simulink library "usask_tlm_lib"  (R2017b)
settings: Solver=ode45  StartTime=0.0  StopTime=10.0  RelTol=1e-3
undefined symbols (not defined in the file or in its folder): B, beta, d, K, L, lambda_1, m_E, m_G, mE_1, mE_2, mG_1, mG_2, nu, r1, r2, rho, T, Zc, Zc_1, Zc_2
libraries: usask_tlm_lib x6, transmission_lines x2
(part 4 of 4)

== system usask_tlm_lib/Tapered TLM Q1P2/G_1 ==
  note: Equation (17) from ven der Buhs et al. 2017
  F + P_1 : Inport
  Sum : Sum  Inputs=+------
  k = 1 : TransferFcn  Numerator=[m_G(1)*T 0]  Denominator=[T n(1)]
  k = 2 : TransferFcn  Numerator=[m_G(2)*T 0]  Denominator=[T n(2)]
  k = 3 : TransferFcn  Numerator=[m_G(3)*T 0]  Denominator=[T n(3)]
  k = 4 : TransferFcn  Numerator=[m_G(4)*T 0]  Denominator=[T n(4)]
  k = 5 : TransferFcn  Numerator=[m_G(5)*T 0]  Denominator=[T n(5)]
  k = 6 : TransferFcn  Numerator=[m_G(6)*T 0]  Denominator=[T n(6)]
  G : Outport
  wires:
  k = 6/1 -> Sum/7
  k = 5/1 -> Sum/6
  k = 4/1 -> Sum/5
  k = 2/1 -> Sum/3
  k = 1/1 -> Sum/2
  k = 3/1 -> Sum/4
  F + P_1/1 -> k = 3/1, k = 2/1, Sum/1, k = 1/1, k = 5/1, k = 6/1, k = 4/1
  Sum/1 -> G/1

== system usask_tlm_lib/Tapered TLM Q1P2/G_2 ==
  note: Equation (17) from ven der Buhs et al. 2017
  F + P_2 : Inport
  Sum : Sum  Inputs=+------
  k = 1 : TransferFcn  Numerator=[m_G(1)*T 0]  Denominator=[T n(1)]
  k = 2 : TransferFcn  Numerator=[m_G(2)*T 0]  Denominator=[T n(2)]
  k = 3 : TransferFcn  Numerator=[m_G(3)*T 0]  Denominator=[T n(3)]
  k = 4 : TransferFcn  Numerator=[m_G(4)*T 0]  Denominator=[T n(4)]
  k = 5 : TransferFcn  Numerator=[m_G(5)*T 0]  Denominator=[T n(5)]
  k = 6 : TransferFcn  Numerator=[m_G(6)*T 0]  Denominator=[T n(6)]
  G : Outport
  wires:
  k = 6/1 -> Sum/7
  k = 5/1 -> Sum/6
  k = 4/1 -> Sum/5
  k = 2/1 -> Sum/3
  k = 1/1 -> Sum/2
  k = 3/1 -> Sum/4
  F + P_2/1 -> k = 3/1, k = 2/1, Sum/1, k = 1/1, k = 5/1, k = 6/1, k = 4/1
  Sum/1 -> G/1

== system usask_tlm_lib/Tapered TLM Q1Q2/  Delay_2  ==
  G : Inport
  Transport Delay : TransportDelay  DelayTime=T_prime
  delay : Outport
  wires:
  Transport Delay/1 -> delay/1
  G/1 -> Transport Delay/1

== system usask_tlm_lib/Tapered TLM Q1Q2/Delay_1  ==
  G : Inport
  Transport Delay : TransportDelay  DelayTime=T_prime
  delay : Outport
  wires:
  Transport Delay/1 -> delay/1
  G/1 -> Transport Delay/1

== system usask_tlm_lib/Tapered TLM Q1Q2/E_1 ==
  note: Equation (14) from ven der Buhs et al. 2017
  Q_1 : Inport
  Gain : Gain  Gain=Z_c
  Sum : Sum  Inputs=++++++
  k = 1 : TransferFcn  Numerator=[m_E(1)]  Denominator=[T n(1)]
  k = 2 : TransferFcn  Numerator=[m_E(2)]  Denominator=[T n(2)]
  k = 3 : TransferFcn  Numerator=[m_E(3)]  Denominator=[T n(3)]
  k = 4 : TransferFcn  Numerator=[m_E(4)]  Denominator=[T n(4)]
  k = 5 : TransferFcn  Numerator=[m_E(5)]  Denominator=[T n(5)]
  k = 6 : TransferFcn  Numerator=[m_E(6)]  Denominator=[T n(6)]
  E : Outport
  wires:
  Q_1/1 -> k = 4/1, k = 5/1, k = 6/1, k = 3/1, k = 1/1, k = 2/1
  k = 6/1 -> Sum/6
  k = 5/1 -> Sum/5
  k = 4/1 -> Sum/4
  k = 3/1 -> Sum/3
  k = 2/1 -> Sum/2
  k = 1/1 -> Sum/1
  Sum/1 -> Gain/1
  Gain/1 -> E/1

== system usask_tlm_lib/Tapered TLM Q1Q2/E_2 ==
  note: Equation (14) from ven der Buhs et al. 2017
  Q_2 : Inport
  Gain : Gain  Gain=Z_c
  Sum : Sum  Inputs=++++++
  k = 1 : TransferFcn  Numerator=[m_E(1)]  Denominator=[T n(1)]
  k = 2 : TransferFcn  Numerator=[m_E(2)]  Denominator=[T n(2)]
  k = 3 : TransferFcn  Numerator=[m_E(3)]  Denominator=[T n(3)]
  k = 4 : TransferFcn  Numerator=[m_E(4)]  Denominator=[T n(4)]
  k = 5 : TransferFcn  Numerator=[m_E(5)]  Denominator=[T n(5)]
  k = 6 : TransferFcn  Numerator=[m_E(6)]  Denominator=[T n(6)]
  E : Outport
  wires:
  Q_2/1 -> k = 4/1, k = 5/1, k = 6/1, k = 3/1, k = 1/1, k = 2/1
  k = 6/1 -> Sum/6
  k = 5/1 -> Sum/5
  k = 4/1 -> Sum/4
  k = 3/1 -> Sum/3
  k = 2/1 -> Sum/2
  k = 1/1 -> Sum/1
  Sum/1 -> Gain/1
  Gain/1 -> E/1

== system usask_tlm_lib/Tapered TLM Q1Q2/F_1 ==
  note: Equation (15) from ven der Buhs et al. 2017
  Q_1 : Inport
  E : Inport  Port=2
  Gain : Gain  Gain=b
  Gain1 : Gain  Gain=Z_c
  Sum : Sum
  F : Outport
  wires:
  E/1 -> Gain/1
  Q_1/1 -> Gain1/1
  Sum/1 -> F/1
  Gain1/1 -> Sum/1
  Gain/1 -> Sum/2

== system usask_tlm_lib/Tapered TLM Q1Q2/F_2 ==
  note: Equation (15) from ven der Buhs et al. 2017
  E : Inport
  Q_2 : Inport  Port=2
  Gain : Gain  Gain=b
  Gain1 : Gain  Gain=Z_c
  Sum : Sum
  F : Outport
  wires:
  Gain/1 -> Sum/2
  Gain1/1 -> Sum/1
  Sum/1 -> F/1
  Q_2/1 -> Gain1/1
  E/1 -> Gain/1

== system usask_tlm_lib/Tapered TLM Q1Q2/G_1 ==
  note: Equation (17) from ven der Buhs et al. 2017
  F + P_1 : Inport
  Sum : Sum  Inputs=+------
  k = 1 : TransferFcn  Numerator=[m_G(1)*T 0]  Denominator=[T n(1)]
  k = 2 : TransferFcn  Numerator=[m_G(2)*T 0]  Denominator=[T n(2)]
  k = 3 : TransferFcn  Numerator=[m_G(3)*T 0]  Denominator=[T n(3)]
  k = 4 : TransferFcn  Numerator=[m_G(4)*T 0]  Denominator=[T n(4)]
  k = 5 : TransferFcn  Numerator=[m_G(5)*T 0]  Denominator=[T n(5)]
  k = 6 : TransferFcn  Numerator=[m_G(6)*T 0]  Denominator=[T n(6)]
  G : Outport
  wires:
  k = 6/1 -> Sum/7
  k = 5/1 -> Sum/6
  k = 4/1 -> Sum/5
  k = 2/1 -> Sum/3
  k = 1/1 -> Sum/2
  k = 3/1 -> Sum/4
  F + P_1/1 -> k = 3/1, k = 2/1, Sum/1, k = 1/1, k = 5/1, k = 6/1, k = 4/1
  Sum/1 -> G/1

== system usask_tlm_lib/Tapered TLM Q1Q2/G_2 ==
  note: Equation (17) from ven der Buhs et al. 2017
  F + P_2 : Inport
  Sum : Sum  Inputs=+------
  k = 1 : TransferFcn  Numerator=[m_G(1)*T 0]  Denominator=[T n(1)]
  k = 2 : TransferFcn  Numerator=[m_G(2)*T 0]  Denominator=[T n(2)]
  k = 3 : TransferFcn  Numerator=[m_G(3)*T 0]  Denominator=[T n(3)]
  k = 4 : TransferFcn  Numerator=[m_G(4)*T 0]  Denominator=[T n(4)]
  k = 5 : TransferFcn  Numerator=[m_G(5)*T 0]  Denominator=[T n(5)]
  k = 6 : TransferFcn  Numerator=[m_G(6)*T 0]  Denominator=[T n(6)]
  G : Outport
  wires:
  k = 6/1 -> Sum/7
  k = 5/1 -> Sum/6
  k = 4/1 -> Sum/5
  k = 2/1 -> Sum/3
  k = 1/1 -> Sum/2
  k = 3/1 -> Sum/4
  F + P_2/1 -> k = 3/1, k = 2/1, Sum/1, k = 1/1, k = 5/1, k = 6/1, k = 4/1
  Sum/1 -> G/1

== system usask_tlm_lib/Internal Blocks/Tapered TLM Base/Delay_1  ==
  G : Inport
  Transport Delay : TransportDelay  DelayTime=T
  delay : Outport
  wires:
  G/1 -> Transport Delay/1
  Transport Delay/1 -> delay/1

== system usask_tlm_lib/Internal Blocks/Tapered TLM Base/Delay_1 1 ==
  G : Inport
  Transport Delay : TransportDelay  DelayTime=T
  delay : Outport
  wires:
  G/1 -> Transport Delay/1
  Transport Delay/1 -> delay/1

== system usask_tlm_lib/Internal Blocks/Tapered TLM Base/E_1 ==
  Q_2 : Inport
  Gain : Gain  Gain=Zc
  Sum : Sum  Inputs=++++++
  k = 1 : TransferFcn  Numerator=[m_E(1)]  Denominator=[T n(1)]
  k = 2 : TransferFcn  Numerator=[m_E(2)]  Denominator=[T n(2)]
  k = 3 : TransferFcn  Numerator=[m_E(3)]  Denominator=[T n(3)]
  k = 4 : TransferFcn  Numerator=[m_E(4)]  Denominator=[T n(4)]
  k = 5 : TransferFcn  Numerator=[m_E(5)]  Denominator=[T n(5)]
  k = 6 : TransferFcn  Numerator=[m_E(6)]  Denominator=[T n(6)]
  E : Outport
  wires:
  Gain/1 -> E/1
  Sum/1 -> Gain/1
  k = 1/1 -> Sum/1
  k = 2/1 -> Sum/2
  k = 3/1 -> Sum/3
  k = 4/1 -> Sum/4
  k = 5/1 -> Sum/5
  k = 6/1 -> Sum/6
  Q_2/1 -> k = 2/1, k = 1/1, k = 3/1, k = 6/1, k = 5/1, k = 4/1

== system usask_tlm_lib/Internal Blocks/Tapered TLM Base/E_2 ==
  Q_2 : Inport
  Gain : Gain  Gain=Zc
  Sum : Sum  Inputs=++++++
  k = 1 : TransferFcn  Numerator=[m_E(1)]  Denominator=[T n(1)]
  k = 2 : TransferFcn  Numerator=[m_E(2)]  Denominator=[T n(2)]
  k = 3 : TransferFcn  Numerator=[m_E(3)]  Denominator=[T n(3)]
  k = 4 : TransferFcn  Numerator=[m_E(4)]  Denominator=[T n(4)]
  k = 5 : TransferFcn  Numerator=[m_E(5)]  Denominator=[T n(5)]
  k = 6 : TransferFcn  Numerator=[m_E(6)]  Denominator=[T n(6)]
  E : Outport
  wires:
  Gain/1 -> E/1
  Sum/1 -> Gain/1
  k = 1/1 -> Sum/1
  k = 2/1 -> Sum/2
  k = 3/1 -> Sum/3
  k = 4/1 -> Sum/4
  k = 5/1 -> Sum/5
  k = 6/1 -> Sum/6
  Q_2/1 -> k = 2/1, k = 1/1, k = 3/1, k = 6/1, k = 5/1, k = 4/1

== system usask_tlm_lib/Internal Blocks/Tapered TLM Base/F_3 ==
  Q_1 : Inport
  E : Inport  Port=2
  Gain : Gain  Gain=b
  Gain1 : Gain  Gain=Zc
  Gain2 : Gain  Gain=F_k
  Sum : Sum
  F : Outport
  wires:
  E/1 -> Gain/1
  Q_1/1 -> Gain1/1
  Sum/1 -> Gain2/1
  Gain1/1 -> Sum/1
  Gain/1 -> Sum/2
  Gain2/1 -> F/1

== system usask_tlm_lib/Internal Blocks/Tapered TLM Base/G_1 ==
  F + P_1 : Inport
  Gain : Gain  Gain=1-H_DC
  Sum : Sum  Inputs=+------
  k = 1 : TransferFcn  Numerator=[m_G(1)*T 0]  Denominator=[T n(1)]
  k = 2 : TransferFcn  Numerator=[m_G(2)*T 0]  Denominator=[T n(2)]
  k = 3 : TransferFcn  Numerator=[m_G(3)*T 0]  Denominator=[T n(3)]
  k = 4 : TransferFcn  Numerator=[m_G(4)*T 0]  Denominator=[T n(4)]
  k = 5 : TransferFcn  Numerator=[m_G(5)*T 0]  Denominator=[T n(5)]
  k = 6 : TransferFcn  Numerator=[m_G(6)*T 0]  Denominator=[T n(6)]
  G : Outport
  wires:
  Sum/1 -> Gain/1
  F + P_1/1 -> k = 4/1, k = 6/1, k = 5/1, k = 1/1, Sum/1, k = 2/1, k = 3/1
  k = 3/1 -> Sum/4
  k = 1/1 -> Sum/2
  k = 2/1 -> Sum/3
  k = 4/1 -> Sum/5
  k = 5/1 -> Sum/6
  k = 6/1 -> Sum/7
  Gain/1 -> G/1

== system usask_tlm_lib/Internal Blocks/Tapered TLM Base/G_3 ==
  F + P_1 : Inport
  Gain : Gain  Gain=1-H_DC
  Sum : Sum  Inputs=+------
  k = 1 : TransferFcn  Numerator=[m_G(1)*T 0]  Denominator=[T n(1)]
  k = 2 : TransferFcn  Numerator=[m_G(2)*T 0]  Denominator=[T n(2)]
  k = 3 : TransferFcn  Numerator=[m_G(3)*T 0]  Denominator=[T n(3)]
  k = 4 : TransferFcn  Numerator=[m_G(4)*T 0]  Denominator=[T n(4)]
  k = 5 : TransferFcn  Numerator=[m_G(5)*T 0]  Denominator=[T n(5)]
  k = 6 : TransferFcn  Numerator=[m_G(6)*T 0]  Denominator=[T n(6)]
  G : Outport
  wires:
  Sum/1 -> Gain/1
  F + P_1/1 -> k = 4/1, k = 6/1, k = 5/1, k = 1/1, Sum/1, k = 2/1, k = 3/1
  k = 3/1 -> Sum/4
  k = 1/1 -> Sum/2
  k = 2/1 -> Sum/3
  k = 4/1 -> Sum/5
  k = 5/1 -> Sum/6
  k = 6/1 -> Sum/7
  Gain/1 -> G/1

== system usask_tlm_lib/Internal Blocks/Tapered TLM Base/H_1 ==
  in : Inport
  Add1 : Sum  Inputs=+-+
  Add2 : Sum  Inputs=-+
  Gain2 : Gain  Gain=H_a
  Gain3 : Gain  Gain=H_b
  Gain5 : Gain  Gain=(H_b-H_a)/T
  Integrator1 : Integrator
  Integrator2 : Integrator
  Integrator3 : Integrator
  Transport Delay1 : TransportDelay  DelayTime=T
  out : Outport
  wires:
  Add2/1 -> Gain5/1
  Integrator1/1 -> Add2/1
  Gain5/1 -> Add1/3
  Gain3/1 -> Add1/2
  Add1/1 -> out/1  "S"
  Gain2/1 -> Add1/1
  Transport Delay1/1 -> Gain3/1, Integrator1/1
  Integrator3/1 -> Add2/2
  Integrator2/1 -> Transport Delay1/1, Gain2/1, Integrator3/1
  in/1 -> Integrator2/1

== system usask_tlm_lib/Internal Blocks/Tapered TLM Base/H_2 ==
  in : Inport
  Add1 : Sum  Inputs=+-+
  Add2 : Sum  Inputs=-+
  Gain2 : Gain  Gain=H_a
  Gain3 : Gain  Gain=H_b
  Gain5 : Gain  Gain=(H_b-H_a)/T
  Integrator1 : Integrator
  Integrator2 : Integrator
  Integrator3 : Integrator
  Transport Delay1 : TransportDelay  DelayTime=T
  out : Outport
  wires:
  Add2/1 -> Gain5/1
  Integrator1/1 -> Add2/1
  Gain5/1 -> Add1/3
  Gain3/1 -> Add1/2
  Add1/1 -> out/1  "S"
  Gain2/1 -> Add1/1
  Transport Delay1/1 -> Gain3/1, Integrator1/1
  Integrator3/1 -> Add2/2
  Integrator2/1 -> Transport Delay1/1, Gain2/1, Integrator3/1
  in/1 -> Integrator2/1

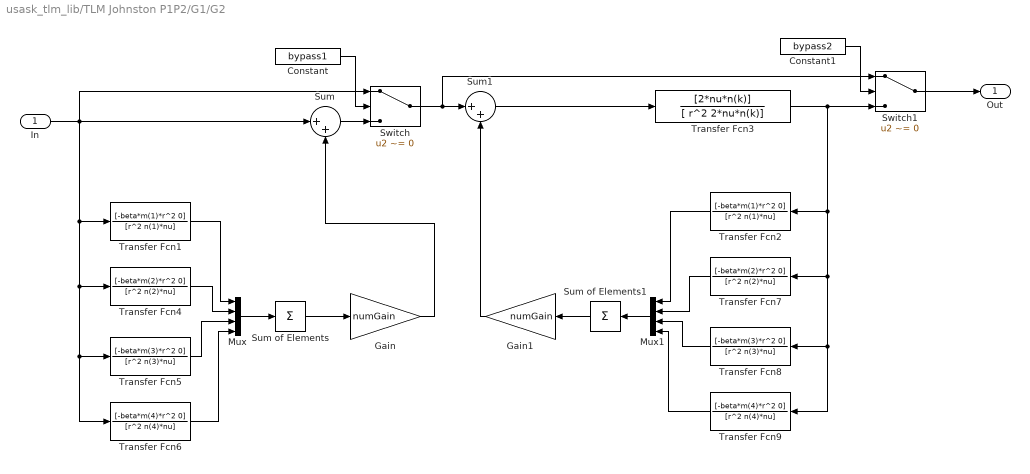
== system usask_tlm_lib/TLM Johnston P1P2/G1/G2 ==
  In : Inport
  Constant : Constant  Value=bypass1
  Constant1 : Constant  Value=bypass2
  Gain : Gain  Gain=numGain
  Gain1 : Gain  Gain=numGain
  Mux : Mux
  Mux1 : Mux
  Sum : Sum  Inputs=|++
  Sum of Elements : Sum  Inputs=+
  Sum of Elements1 : Sum  Inputs=+
  Sum1 : Sum  Inputs=|++
  Switch : Switch  Criteria=u2 ~= 0
  Switch1 : Switch  Criteria=u2 ~= 0
  Transfer Fcn1 : TransferFcn  Numerator=[-beta*m(1)*r^2 0]  Denominator=[r^2 n(1)*nu]
  Transfer Fcn2 : TransferFcn  Numerator=[-beta*m(1)*r^2 0]  Denominator=[r^2 n(1)*nu]
  Transfer Fcn3 : TransferFcn  Numerator=[2*nu*n(k)]  Denominator=[ r^2 2*nu*n(k)]
  Transfer Fcn4 : TransferFcn  Numerator=[-beta*m(2)*r^2 0]  Denominator=[r^2 n(2)*nu]
  Transfer Fcn5 : TransferFcn  Numerator=[-beta*m(3)*r^2 0]  Denominator=[r^2 n(3)*nu]
  Transfer Fcn6 : TransferFcn  Numerator=[-beta*m(4)*r^2 0]  Denominator=[r^2 n(4)*nu]
  Transfer Fcn7 : TransferFcn  Numerator=[-beta*m(2)*r^2 0]  Denominator=[r^2 n(2)*nu]
  Transfer Fcn8 : TransferFcn  Numerator=[-beta*m(3)*r^2 0]  Denominator=[r^2 n(3)*nu]
  Transfer Fcn9 : TransferFcn  Numerator=[-beta*m(4)*r^2 0]  Denominator=[r^2 n(4)*nu]
  Out : Outport
  wires:
  Sum1/1 -> Transfer Fcn3/1
  Gain1/1 -> Sum1/2
  Gain/1 -> Sum/2
  Mux1/1 -> Sum of Elements1/1
  Transfer Fcn9/1 -> Mux1/4
  Transfer Fcn2/1 -> Mux1/1
  Transfer Fcn8/1 -> Mux1/3
  Transfer Fcn7/1 -> Mux1/2
  Sum of Elements1/1 -> Gain1/1
  Mux/1 -> Sum of Elements/1
  Transfer Fcn6/1 -> Mux/4
  Transfer Fcn1/1 -> Mux/1
  Transfer Fcn5/1 -> Mux/3
  Transfer Fcn4/1 -> Mux/2
  Constant1/1 -> Switch1/2
  Constant/1 -> Switch/2
  Switch1/1 -> Out/1
  Switch/1 -> Sum1/1, Switch1/1
  Sum/1 -> Switch/3
  Transfer Fcn3/1 -> Switch1/3, Transfer Fcn2/1, Transfer Fcn7/1, Transfer Fcn8/1, Transfer Fcn9/1
  Sum of Elements/1 -> Gain/1
  In/1 -> Sum/1, Transfer Fcn1/1, Transfer Fcn4/1, Transfer Fcn5/1, Transfer Fcn6/1, Switch/1

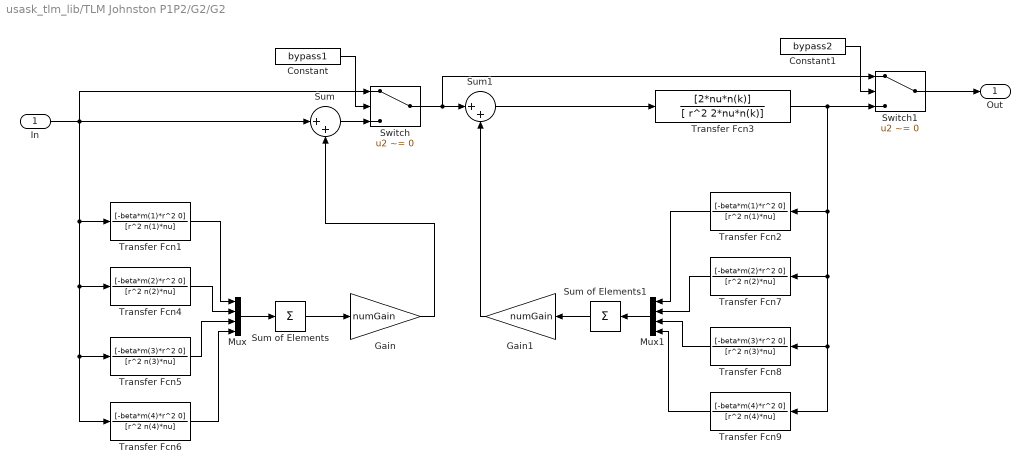
== system usask_tlm_lib/TLM Johnston P1P2/G2/G2 ==
  In : Inport
  Constant : Constant  Value=bypass1
  Constant1 : Constant  Value=bypass2
  Gain : Gain  Gain=numGain
  Gain1 : Gain  Gain=numGain
  Mux : Mux
  Mux1 : Mux
  Sum : Sum  Inputs=|++
  Sum of Elements : Sum  Inputs=+
  Sum of Elements1 : Sum  Inputs=+
  Sum1 : Sum  Inputs=|++
  Switch : Switch  Criteria=u2 ~= 0
  Switch1 : Switch  Criteria=u2 ~= 0
  Transfer Fcn1 : TransferFcn  Numerator=[-beta*m(1)*r^2 0]  Denominator=[r^2 n(1)*nu]
  Transfer Fcn2 : TransferFcn  Numerator=[-beta*m(1)*r^2 0]  Denominator=[r^2 n(1)*nu]
  Transfer Fcn3 : TransferFcn  Numerator=[2*nu*n(k)]  Denominator=[ r^2 2*nu*n(k)]
  Transfer Fcn4 : TransferFcn  Numerator=[-beta*m(2)*r^2 0]  Denominator=[r^2 n(2)*nu]
  Transfer Fcn5 : TransferFcn  Numerator=[-beta*m(3)*r^2 0]  Denominator=[r^2 n(3)*nu]
  Transfer Fcn6 : TransferFcn  Numerator=[-beta*m(4)*r^2 0]  Denominator=[r^2 n(4)*nu]
  Transfer Fcn7 : TransferFcn  Numerator=[-beta*m(2)*r^2 0]  Denominator=[r^2 n(2)*nu]
  Transfer Fcn8 : TransferFcn  Numerator=[-beta*m(3)*r^2 0]  Denominator=[r^2 n(3)*nu]
  Transfer Fcn9 : TransferFcn  Numerator=[-beta*m(4)*r^2 0]  Denominator=[r^2 n(4)*nu]
  Out : Outport
  wires:
  Sum1/1 -> Transfer Fcn3/1
  Gain1/1 -> Sum1/2
  Gain/1 -> Sum/2
  Mux1/1 -> Sum of Elements1/1
  Transfer Fcn9/1 -> Mux1/4
  Transfer Fcn2/1 -> Mux1/1
  Transfer Fcn8/1 -> Mux1/3
  Transfer Fcn7/1 -> Mux1/2
  Sum of Elements1/1 -> Gain1/1
  Mux/1 -> Sum of Elements/1
  Transfer Fcn6/1 -> Mux/4
  Transfer Fcn1/1 -> Mux/1
  Transfer Fcn5/1 -> Mux/3
  Transfer Fcn4/1 -> Mux/2
  Constant1/1 -> Switch1/2
  Constant/1 -> Switch/2
  Switch1/1 -> Out/1
  Switch/1 -> Sum1/1, Switch1/1
  Sum/1 -> Switch/3
  Transfer Fcn3/1 -> Switch1/3, Transfer Fcn2/1, Transfer Fcn7/1, Transfer Fcn8/1, Transfer Fcn9/1
  Sum of Elements/1 -> Gain/1
  In/1 -> Sum/1, Transfer Fcn1/1, Transfer Fcn4/1, Transfer Fcn5/1, Transfer Fcn6/1, Switch/1

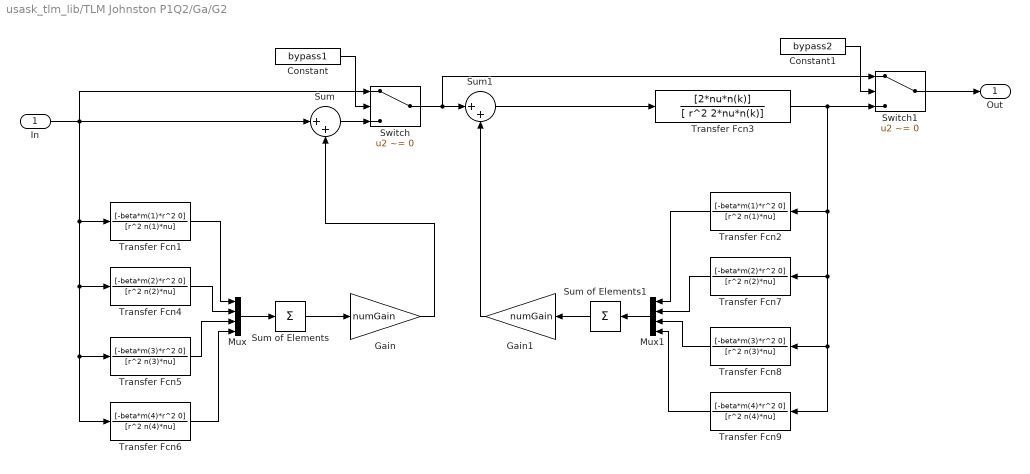
== system usask_tlm_lib/TLM Johnston P1Q2/Ga/G2 ==
  In : Inport
  Constant : Constant  Value=bypass1
  Constant1 : Constant  Value=bypass2
  Gain : Gain  Gain=numGain
  Gain1 : Gain  Gain=numGain
  Mux : Mux
  Mux1 : Mux
  Sum : Sum  Inputs=|++
  Sum of Elements : Sum  Inputs=+
  Sum of Elements1 : Sum  Inputs=+
  Sum1 : Sum  Inputs=|++
  Switch : Switch  Criteria=u2 ~= 0
  Switch1 : Switch  Criteria=u2 ~= 0
  Transfer Fcn1 : TransferFcn  Numerator=[-beta*m(1)*r^2 0]  Denominator=[r^2 n(1)*nu]
  Transfer Fcn2 : TransferFcn  Numerator=[-beta*m(1)*r^2 0]  Denominator=[r^2 n(1)*nu]
  Transfer Fcn3 : TransferFcn  Numerator=[2*nu*n(k)]  Denominator=[ r^2 2*nu*n(k)]
  Transfer Fcn4 : TransferFcn  Numerator=[-beta*m(2)*r^2 0]  Denominator=[r^2 n(2)*nu]
  Transfer Fcn5 : TransferFcn  Numerator=[-beta*m(3)*r^2 0]  Denominator=[r^2 n(3)*nu]
  Transfer Fcn6 : TransferFcn  Numerator=[-beta*m(4)*r^2 0]  Denominator=[r^2 n(4)*nu]
  Transfer Fcn7 : TransferFcn  Numerator=[-beta*m(2)*r^2 0]  Denominator=[r^2 n(2)*nu]
  Transfer Fcn8 : TransferFcn  Numerator=[-beta*m(3)*r^2 0]  Denominator=[r^2 n(3)*nu]
  Transfer Fcn9 : TransferFcn  Numerator=[-beta*m(4)*r^2 0]  Denominator=[r^2 n(4)*nu]
  Out : Outport
  wires:
  In/1 -> Switch/1, Transfer Fcn6/1, Transfer Fcn5/1, Transfer Fcn4/1, Transfer Fcn1/1, Sum/1
  Sum of Elements/1 -> Gain/1
  Transfer Fcn3/1 -> Transfer Fcn9/1, Transfer Fcn8/1, Transfer Fcn7/1, Transfer Fcn2/1, Switch1/3
  Sum/1 -> Switch/3
  Switch/1 -> Switch1/1, Sum1/1
  Switch1/1 -> Out/1
  Constant/1 -> Switch/2
  Constant1/1 -> Switch1/2
  Transfer Fcn4/1 -> Mux/2
  Transfer Fcn5/1 -> Mux/3
  Transfer Fcn1/1 -> Mux/1
  Transfer Fcn6/1 -> Mux/4
  Mux/1 -> Sum of Elements/1
  Sum of Elements1/1 -> Gain1/1
  Transfer Fcn7/1 -> Mux1/2
  Transfer Fcn8/1 -> Mux1/3
  Transfer Fcn2/1 -> Mux1/1
  Transfer Fcn9/1 -> Mux1/4
  Mux1/1 -> Sum of Elements1/1
  Gain/1 -> Sum/2
  Gain1/1 -> Sum1/2
  Sum1/1 -> Transfer Fcn3/1

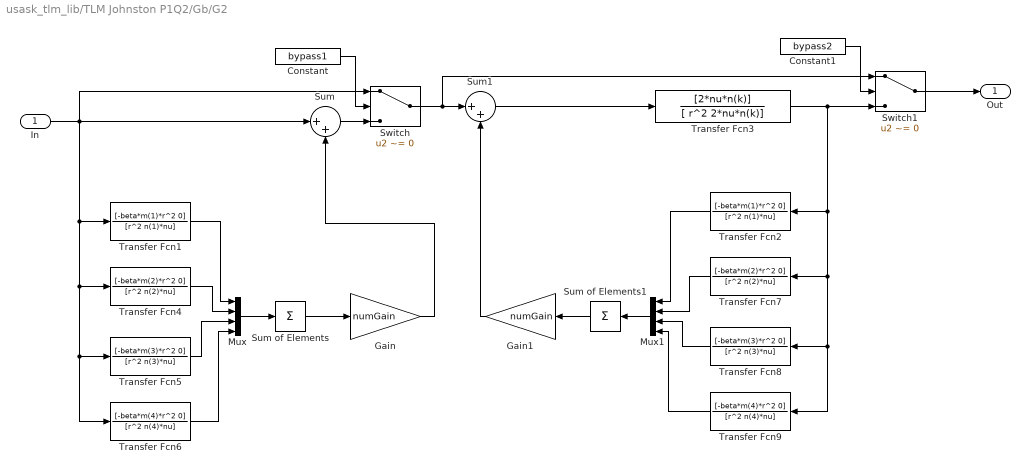
== system usask_tlm_lib/TLM Johnston P1Q2/Gb/G2 ==
  In : Inport
  Constant : Constant  Value=bypass1
  Constant1 : Constant  Value=bypass2
  Gain : Gain  Gain=numGain
  Gain1 : Gain  Gain=numGain
  Mux : Mux
  Mux1 : Mux
  Sum : Sum  Inputs=|++
  Sum of Elements : Sum  Inputs=+
  Sum of Elements1 : Sum  Inputs=+
  Sum1 : Sum  Inputs=|++
  Switch : Switch  Criteria=u2 ~= 0
  Switch1 : Switch  Criteria=u2 ~= 0
  Transfer Fcn1 : TransferFcn  Numerator=[-beta*m(1)*r^2 0]  Denominator=[r^2 n(1)*nu]
  Transfer Fcn2 : TransferFcn  Numerator=[-beta*m(1)*r^2 0]  Denominator=[r^2 n(1)*nu]
  Transfer Fcn3 : TransferFcn  Numerator=[2*nu*n(k)]  Denominator=[ r^2 2*nu*n(k)]
  Transfer Fcn4 : TransferFcn  Numerator=[-beta*m(2)*r^2 0]  Denominator=[r^2 n(2)*nu]
  Transfer Fcn5 : TransferFcn  Numerator=[-beta*m(3)*r^2 0]  Denominator=[r^2 n(3)*nu]
  Transfer Fcn6 : TransferFcn  Numerator=[-beta*m(4)*r^2 0]  Denominator=[r^2 n(4)*nu]
  Transfer Fcn7 : TransferFcn  Numerator=[-beta*m(2)*r^2 0]  Denominator=[r^2 n(2)*nu]
  Transfer Fcn8 : TransferFcn  Numerator=[-beta*m(3)*r^2 0]  Denominator=[r^2 n(3)*nu]
  Transfer Fcn9 : TransferFcn  Numerator=[-beta*m(4)*r^2 0]  Denominator=[r^2 n(4)*nu]
  Out : Outport
  wires:
  In/1 -> Switch/1, Transfer Fcn6/1, Transfer Fcn5/1, Transfer Fcn4/1, Transfer Fcn1/1, Sum/1
  Sum of Elements/1 -> Gain/1
  Transfer Fcn3/1 -> Transfer Fcn9/1, Transfer Fcn8/1, Transfer Fcn7/1, Transfer Fcn2/1, Switch1/3
  Sum/1 -> Switch/3
  Switch/1 -> Switch1/1, Sum1/1
  Switch1/1 -> Out/1
  Constant/1 -> Switch/2
  Constant1/1 -> Switch1/2
  Transfer Fcn4/1 -> Mux/2
  Transfer Fcn5/1 -> Mux/3
  Transfer Fcn1/1 -> Mux/1
  Transfer Fcn6/1 -> Mux/4
  Mux/1 -> Sum of Elements/1
  Sum of Elements1/1 -> Gain1/1
  Transfer Fcn7/1 -> Mux1/2
  Transfer Fcn8/1 -> Mux1/3
  Transfer Fcn2/1 -> Mux1/1
  Transfer Fcn9/1 -> Mux1/4
  Mux1/1 -> Sum of Elements1/1
  Gain/1 -> Sum/2
  Gain1/1 -> Sum1/2
  Sum1/1 -> Transfer Fcn3/1

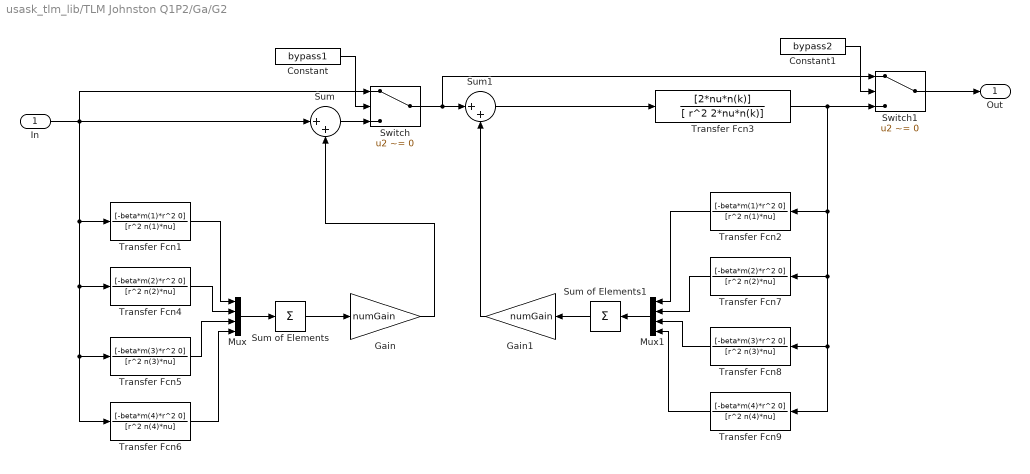
== system usask_tlm_lib/TLM Johnston Q1P2/Ga/G2 ==
  In : Inport
  Constant : Constant  Value=bypass1
  Constant1 : Constant  Value=bypass2
  Gain : Gain  Gain=numGain
  Gain1 : Gain  Gain=numGain
  Mux : Mux
  Mux1 : Mux
  Sum : Sum  Inputs=|++
  Sum of Elements : Sum  Inputs=+
  Sum of Elements1 : Sum  Inputs=+
  Sum1 : Sum  Inputs=|++
  Switch : Switch  Criteria=u2 ~= 0
  Switch1 : Switch  Criteria=u2 ~= 0
  Transfer Fcn1 : TransferFcn  Numerator=[-beta*m(1)*r^2 0]  Denominator=[r^2 n(1)*nu]
  Transfer Fcn2 : TransferFcn  Numerator=[-beta*m(1)*r^2 0]  Denominator=[r^2 n(1)*nu]
  Transfer Fcn3 : TransferFcn  Numerator=[2*nu*n(k)]  Denominator=[ r^2 2*nu*n(k)]
  Transfer Fcn4 : TransferFcn  Numerator=[-beta*m(2)*r^2 0]  Denominator=[r^2 n(2)*nu]
  Transfer Fcn5 : TransferFcn  Numerator=[-beta*m(3)*r^2 0]  Denominator=[r^2 n(3)*nu]
  Transfer Fcn6 : TransferFcn  Numerator=[-beta*m(4)*r^2 0]  Denominator=[r^2 n(4)*nu]
  Transfer Fcn7 : TransferFcn  Numerator=[-beta*m(2)*r^2 0]  Denominator=[r^2 n(2)*nu]
  Transfer Fcn8 : TransferFcn  Numerator=[-beta*m(3)*r^2 0]  Denominator=[r^2 n(3)*nu]
  Transfer Fcn9 : TransferFcn  Numerator=[-beta*m(4)*r^2 0]  Denominator=[r^2 n(4)*nu]
  Out : Outport
  wires:
  In/1 -> Switch/1, Transfer Fcn6/1, Transfer Fcn5/1, Transfer Fcn4/1, Transfer Fcn1/1, Sum/1
  Sum of Elements/1 -> Gain/1
  Transfer Fcn3/1 -> Transfer Fcn9/1, Transfer Fcn8/1, Transfer Fcn7/1, Transfer Fcn2/1, Switch1/3
  Sum/1 -> Switch/3
  Switch/1 -> Switch1/1, Sum1/1
  Switch1/1 -> Out/1
  Constant/1 -> Switch/2
  Constant1/1 -> Switch1/2
  Transfer Fcn4/1 -> Mux/2
  Transfer Fcn5/1 -> Mux/3
  Transfer Fcn1/1 -> Mux/1
  Transfer Fcn6/1 -> Mux/4
  Mux/1 -> Sum of Elements/1
  Sum of Elements1/1 -> Gain1/1
  Transfer Fcn7/1 -> Mux1/2
  Transfer Fcn8/1 -> Mux1/3
  Transfer Fcn2/1 -> Mux1/1
  Transfer Fcn9/1 -> Mux1/4
  Mux1/1 -> Sum of Elements1/1
  Gain/1 -> Sum/2
  Gain1/1 -> Sum1/2
  Sum1/1 -> Transfer Fcn3/1

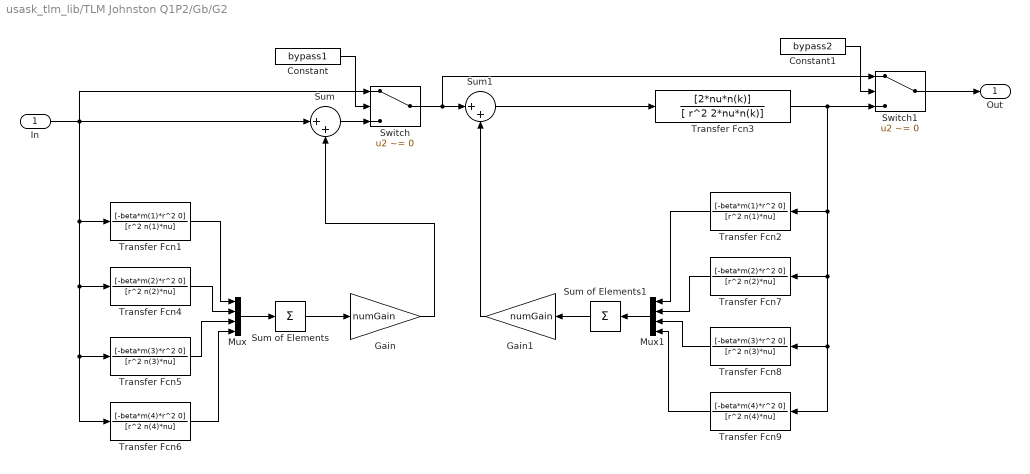
== system usask_tlm_lib/TLM Johnston Q1P2/Gb/G2 ==
  In : Inport
  Constant : Constant  Value=bypass1
  Constant1 : Constant  Value=bypass2
  Gain : Gain  Gain=numGain
  Gain1 : Gain  Gain=numGain
  Mux : Mux
  Mux1 : Mux
  Sum : Sum  Inputs=|++
  Sum of Elements : Sum  Inputs=+
  Sum of Elements1 : Sum  Inputs=+
  Sum1 : Sum  Inputs=|++
  Switch : Switch  Criteria=u2 ~= 0
  Switch1 : Switch  Criteria=u2 ~= 0
  Transfer Fcn1 : TransferFcn  Numerator=[-beta*m(1)*r^2 0]  Denominator=[r^2 n(1)*nu]
  Transfer Fcn2 : TransferFcn  Numerator=[-beta*m(1)*r^2 0]  Denominator=[r^2 n(1)*nu]
  Transfer Fcn3 : TransferFcn  Numerator=[2*nu*n(k)]  Denominator=[ r^2 2*nu*n(k)]
  Transfer Fcn4 : TransferFcn  Numerator=[-beta*m(2)*r^2 0]  Denominator=[r^2 n(2)*nu]
  Transfer Fcn5 : TransferFcn  Numerator=[-beta*m(3)*r^2 0]  Denominator=[r^2 n(3)*nu]
  Transfer Fcn6 : TransferFcn  Numerator=[-beta*m(4)*r^2 0]  Denominator=[r^2 n(4)*nu]
  Transfer Fcn7 : TransferFcn  Numerator=[-beta*m(2)*r^2 0]  Denominator=[r^2 n(2)*nu]
  Transfer Fcn8 : TransferFcn  Numerator=[-beta*m(3)*r^2 0]  Denominator=[r^2 n(3)*nu]
  Transfer Fcn9 : TransferFcn  Numerator=[-beta*m(4)*r^2 0]  Denominator=[r^2 n(4)*nu]
  Out : Outport
  wires:
  In/1 -> Switch/1, Transfer Fcn6/1, Transfer Fcn5/1, Transfer Fcn4/1, Transfer Fcn1/1, Sum/1
  Sum of Elements/1 -> Gain/1
  Transfer Fcn3/1 -> Transfer Fcn9/1, Transfer Fcn8/1, Transfer Fcn7/1, Transfer Fcn2/1, Switch1/3
  Sum/1 -> Switch/3
  Switch/1 -> Switch1/1, Sum1/1
  Switch1/1 -> Out/1
  Constant/1 -> Switch/2
  Constant1/1 -> Switch1/2
  Transfer Fcn4/1 -> Mux/2
  Transfer Fcn5/1 -> Mux/3
  Transfer Fcn1/1 -> Mux/1
  Transfer Fcn6/1 -> Mux/4
  Mux/1 -> Sum of Elements/1
  Sum of Elements1/1 -> Gain1/1
  Transfer Fcn7/1 -> Mux1/2
  Transfer Fcn8/1 -> Mux1/3
  Transfer Fcn2/1 -> Mux1/1
  Transfer Fcn9/1 -> Mux1/4
  Mux1/1 -> Sum of Elements1/1
  Gain/1 -> Sum/2
  Gain1/1 -> Sum1/2
  Sum1/1 -> Transfer Fcn3/1

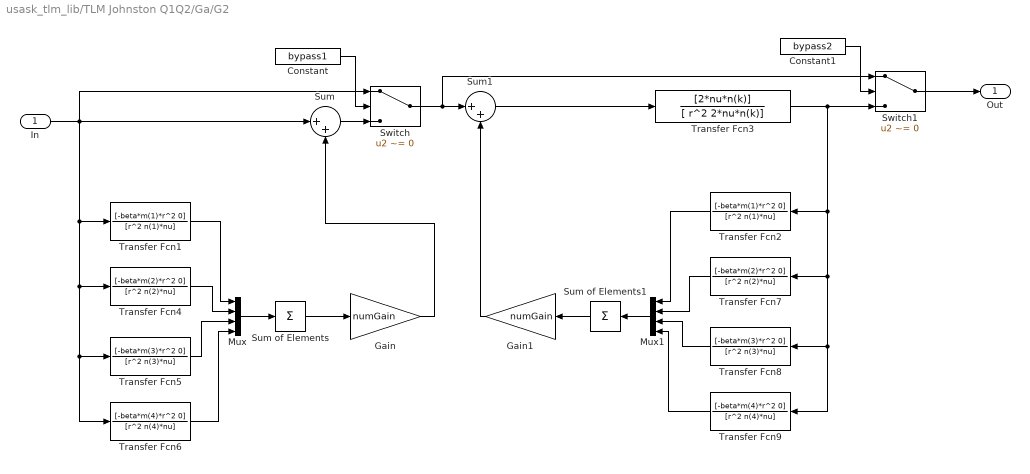
== system usask_tlm_lib/TLM Johnston Q1Q2/Ga/G2 ==
  In : Inport
  Constant : Constant  Value=bypass1
  Constant1 : Constant  Value=bypass2
  Gain : Gain  Gain=numGain
  Gain1 : Gain  Gain=numGain
  Mux : Mux
  Mux1 : Mux
  Sum : Sum  Inputs=|++
  Sum of Elements : Sum  Inputs=+
  Sum of Elements1 : Sum  Inputs=+
  Sum1 : Sum  Inputs=|++
  Switch : Switch  Criteria=u2 ~= 0
  Switch1 : Switch  Criteria=u2 ~= 0
  Transfer Fcn1 : TransferFcn  Numerator=[-beta*m(1)*r^2 0]  Denominator=[r^2 n(1)*nu]
  Transfer Fcn2 : TransferFcn  Numerator=[-beta*m(1)*r^2 0]  Denominator=[r^2 n(1)*nu]
  Transfer Fcn3 : TransferFcn  Numerator=[2*nu*n(k)]  Denominator=[ r^2 2*nu*n(k)]
  Transfer Fcn4 : TransferFcn  Numerator=[-beta*m(2)*r^2 0]  Denominator=[r^2 n(2)*nu]
  Transfer Fcn5 : TransferFcn  Numerator=[-beta*m(3)*r^2 0]  Denominator=[r^2 n(3)*nu]
  Transfer Fcn6 : TransferFcn  Numerator=[-beta*m(4)*r^2 0]  Denominator=[r^2 n(4)*nu]
  Transfer Fcn7 : TransferFcn  Numerator=[-beta*m(2)*r^2 0]  Denominator=[r^2 n(2)*nu]
  Transfer Fcn8 : TransferFcn  Numerator=[-beta*m(3)*r^2 0]  Denominator=[r^2 n(3)*nu]
  Transfer Fcn9 : TransferFcn  Numerator=[-beta*m(4)*r^2 0]  Denominator=[r^2 n(4)*nu]
  Out : Outport
  wires:
  In/1 -> Switch/1, Transfer Fcn6/1, Transfer Fcn5/1, Transfer Fcn4/1, Transfer Fcn1/1, Sum/1
  Sum of Elements/1 -> Gain/1
  Transfer Fcn3/1 -> Transfer Fcn9/1, Transfer Fcn8/1, Transfer Fcn7/1, Transfer Fcn2/1, Switch1/3
  Sum/1 -> Switch/3
  Switch/1 -> Switch1/1, Sum1/1
  Switch1/1 -> Out/1
  Constant/1 -> Switch/2
  Constant1/1 -> Switch1/2
  Transfer Fcn4/1 -> Mux/2
  Transfer Fcn5/1 -> Mux/3
  Transfer Fcn1/1 -> Mux/1
  Transfer Fcn6/1 -> Mux/4
  Mux/1 -> Sum of Elements/1
  Sum of Elements1/1 -> Gain1/1
  Transfer Fcn7/1 -> Mux1/2
  Transfer Fcn8/1 -> Mux1/3
  Transfer Fcn2/1 -> Mux1/1
  Transfer Fcn9/1 -> Mux1/4
  Mux1/1 -> Sum of Elements1/1
  Gain/1 -> Sum/2
  Gain1/1 -> Sum1/2
  Sum1/1 -> Transfer Fcn3/1

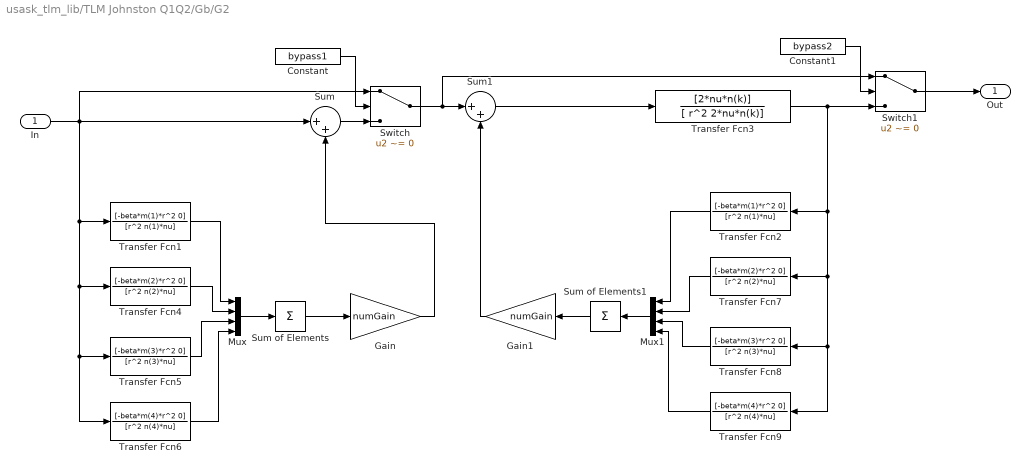
== system usask_tlm_lib/TLM Johnston Q1Q2/Gb/G2 ==
  In : Inport
  Constant : Constant  Value=bypass1
  Constant1 : Constant  Value=bypass2
  Gain : Gain  Gain=numGain
  Gain1 : Gain  Gain=numGain
  Mux : Mux
  Mux1 : Mux
  Sum : Sum  Inputs=|++
  Sum of Elements : Sum  Inputs=+
  Sum of Elements1 : Sum  Inputs=+
  Sum1 : Sum  Inputs=|++
  Switch : Switch  Criteria=u2 ~= 0
  Switch1 : Switch  Criteria=u2 ~= 0
  Transfer Fcn1 : TransferFcn  Numerator=[-beta*m(1)*r^2 0]  Denominator=[r^2 n(1)*nu]
  Transfer Fcn2 : TransferFcn  Numerator=[-beta*m(1)*r^2 0]  Denominator=[r^2 n(1)*nu]
  Transfer Fcn3 : TransferFcn  Numerator=[2*nu*n(k)]  Denominator=[ r^2 2*nu*n(k)]
  Transfer Fcn4 : TransferFcn  Numerator=[-beta*m(2)*r^2 0]  Denominator=[r^2 n(2)*nu]
  Transfer Fcn5 : TransferFcn  Numerator=[-beta*m(3)*r^2 0]  Denominator=[r^2 n(3)*nu]
  Transfer Fcn6 : TransferFcn  Numerator=[-beta*m(4)*r^2 0]  Denominator=[r^2 n(4)*nu]
  Transfer Fcn7 : TransferFcn  Numerator=[-beta*m(2)*r^2 0]  Denominator=[r^2 n(2)*nu]
  Transfer Fcn8 : TransferFcn  Numerator=[-beta*m(3)*r^2 0]  Denominator=[r^2 n(3)*nu]
  Transfer Fcn9 : TransferFcn  Numerator=[-beta*m(4)*r^2 0]  Denominator=[r^2 n(4)*nu]
  Out : Outport
  wires:
  In/1 -> Switch/1, Transfer Fcn6/1, Transfer Fcn5/1, Transfer Fcn4/1, Transfer Fcn1/1, Sum/1
  Sum of Elements/1 -> Gain/1
  Transfer Fcn3/1 -> Transfer Fcn9/1, Transfer Fcn8/1, Transfer Fcn7/1, Transfer Fcn2/1, Switch1/3
  Sum/1 -> Switch/3
  Switch/1 -> Switch1/1, Sum1/1
  Switch1/1 -> Out/1
  Constant/1 -> Switch/2
  Constant1/1 -> Switch1/2
  Transfer Fcn4/1 -> Mux/2
  Transfer Fcn5/1 -> Mux/3
  Transfer Fcn1/1 -> Mux/1
  Transfer Fcn6/1 -> Mux/4
  Mux/1 -> Sum of Elements/1
  Sum of Elements1/1 -> Gain1/1
  Transfer Fcn7/1 -> Mux1/2
  Transfer Fcn8/1 -> Mux1/3
  Transfer Fcn2/1 -> Mux1/1
  Transfer Fcn9/1 -> Mux1/4
  Mux1/1 -> Sum of Elements1/1
  Gain/1 -> Sum/2
  Gain1/1 -> Sum1/2
  Sum1/1 -> Transfer Fcn3/1
